simulink model "sync_enable_example"  (R2017b)
settings: Solver=FixedStepDiscrete  StartTime=0.0  StopTime=10.0  RelTol=1e-3
libraries: hdlsllib x2, simulink x1
settings Model: DataTypeOverride=Off  Creator=cchung  LastModifiedBy=jerickso
settings DataIOCC: SaveOutput=off  SaveTime=off
settings OptimizationCC: BlockReduction=off  ConditionallyExecuteInputs=off  DefaultParameterBehavior=Inlined
settings DebuggingCC: AlgebraicLoopMsg=error  SingleTaskRateTransMsg=error  StrictBusMsg=ErrorOnBusTreatedAsVector
settings HardwareCC: ProdBitPerPointer=32  ProdBitPerSizeT=32  ProdBitPerPtrDiffT=32  ProdLargestAtomicFloat=None  ProdIntDivRoundTo=Undefined  ProdEndianess=Unspecified  ProdWordSize=32  ProdHWDeviceType=ASIC/FPGA->ASIC/FPGA  ProdEqTarget=off
settings CodeAppCC: StateflowObjectComments=on

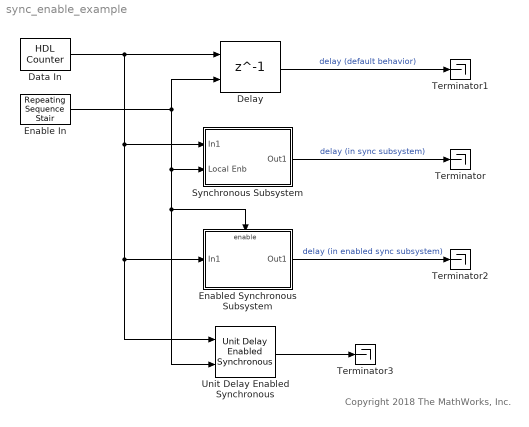
== system sync_enable_example ==
  note: Copyright 2018 The MathWorks, Inc.
  Data In : hdlsllib/Sources/HDL Counter  CountType=Free running  CountInit=0  CountStep=1  CountMax=25  CountFromType=Initial value  CountFrom=0  CountResetPort=off  CountLoadPort=off  CountEnbPort=off  CountDirPort=off  CountDataType=Unsigned  CountWordLen=8  CountFracLen=0  CountSampTime=1
      settings: SourceProductBaseCode=HD
  Delay : Delay  DelayLength=1  ShowEnablePort=on
      settings: InputPortMap=u0,e6
  Enable In : simulink/Sources/Repeating Sequence Stair  OutValues=[0 1 0 0 1 1 0 0]  tsamp=1  OutMin=[]  OutMax=[]  OutDataTypeStr=fixdt('boolean')  OutputDataTypeScalingMode=Specify via dialog  OutDataType=fixdt('boolean')  ConRadixGroup=Best Precision: Vector-wise  OutScaling=[]
  Enabled Synchronous Subsystem : Subsystem  TreatAsAtomicUnit=on
  Synchronous Subsystem : Subsystem
  Terminator{,1..3} (4 alike) : Terminator
  Unit Delay Enabled Synchronous : hdlsllib/Discrete/Unit Delay Enabled Synchronous  InitialCondition=0.0  SampleTime=-1
      settings: SourceProductName=HDL Coder  SourceProductBaseCode=HD
  wires:
  Data In/1 -> Unit Delay Enabled Synchronous/1, Enabled Synchronous Subsystem/1(In1), Synchronous Subsystem/1(In1), Delay/1
  Synchronous Subsystem/1(Out1) -> Terminator/1  "delay (in sync subsystem)"
  Delay/1 -> Terminator1/1  "delay (default behavior)"
  Enabled Synchronous Subsystem/1(Out1) -> Terminator2/1  "delay (in enabled sync subsystem)"
  Enable In/1 -> Unit Delay Enabled Synchronous/2, Enabled Synchronous Subsystem/Enable, Synchronous Subsystem/2(Local Enb), Delay/2
  Unit Delay Enabled Synchronous/1 -> Terminator3/1

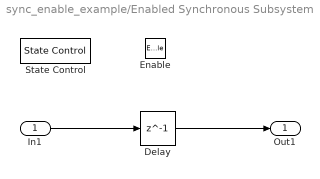
== system sync_enable_example/Enabled Synchronous Subsystem ==
  In1 : Inport
  Enable : EnablePort
  Delay : Delay  DelayLength=1
  State Control : StateControl  StateControl=Synchronous
  Out1 : Outport
  wires:
  In1/1 -> Delay/1
  Delay/1 -> Out1/1

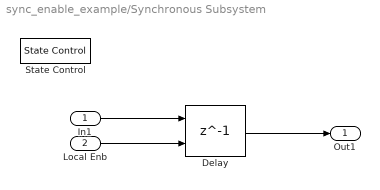
== system sync_enable_example/Synchronous Subsystem ==
  In1 : Inport
  Local Enb : Inport  Port=2
  Delay : Delay  DelayLength=1  ShowEnablePort=on
      settings: InputPortMap=u0,e6
  State Control : StateControl  StateControl=Synchronous
  Out1 : Outport
  wires:
  In1/1 -> Delay/1
  Local Enb/1 -> Delay/2
  Delay/1 -> Out1/1
